simulink model "Salmuera"  (R2021b)
settings: Solver=VariableStepAuto  StartTime=0.0  StopTime=99  RelTol=1e-3
settings Model: Creator=juandiegocastropadilla  LastModifiedBy=juandiegocastropadilla

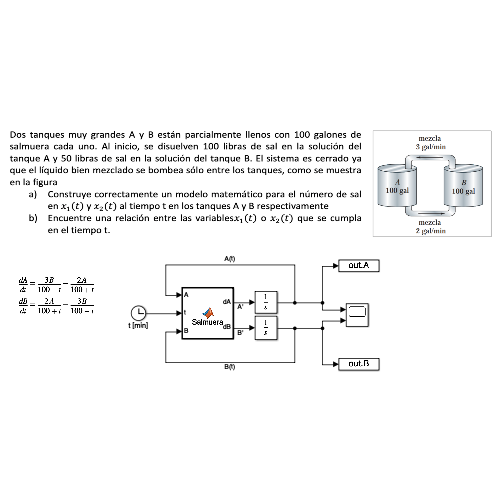
[thumbnail: Simulink's stored preview of the top-level diagram]
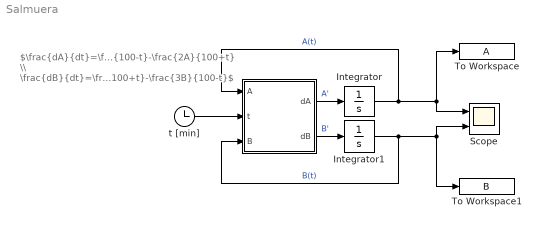
== system Salmuera ==
  note: $\frac{dA}{dt}=\frac{3B}{100-t}-\frac{2A}{100+t} \\ \frac{dB}{dt}=\frac{2A}{100+t}-\frac{3B}{100-t}$
  " " : MATLAB Function  TreatAsAtomicUnit=on
  Integrator : Integrator  InitialCondition=100
  Integrator1 : Integrator  InitialCondition=50
  Scope : Scope  NumInputPorts=2
  To Workspace : ToWorkspace  VariableName=A  SampleTime=-1
  To Workspace1 : ToWorkspace  VariableName=B  SampleTime=-1
  t [min] : Clock
  wires:
  Integrator/1 -> " "/1(A), Scope/1, To Workspace/1  "A(t)"
  " "/1(dA) -> Integrator/1  "A'"
  Integrator1/1 -> " "/3(B), Scope/2, To Workspace1/1  "B(t)"
  " "/2(dB) -> Integrator1/1  "B'"
  t [min]/1 -> " "/2(t)

== matlab function Salmuera/  ==
  data: A input; t input; dA output; B input; dB output
function [dA, dB] = Salmuera(A, t, B)

VA0 = 100; % (gal)
VB0 = 100; % (gal)

R1 = 3; % (gal/min)
R2 = 2; % (gal/min)

VA = VA0 + t*(R1-R2); % (gal)
VB = VB0 + t*(R2-R1); % (gal)

dA = (R1*B)/(VB) - (R2*A)/(VA);
dB = (R2*A)/(VA) - (R1*B)/(VB);
